simulink model "Tarea_1"  (R2013a)
settings: Solver=ode45  StartTime=0.0  StopTime=10  RelTol=1e-3
libraries: simulink x1
settings Model: Creator=Miguel  LastModifiedBy=Miguel

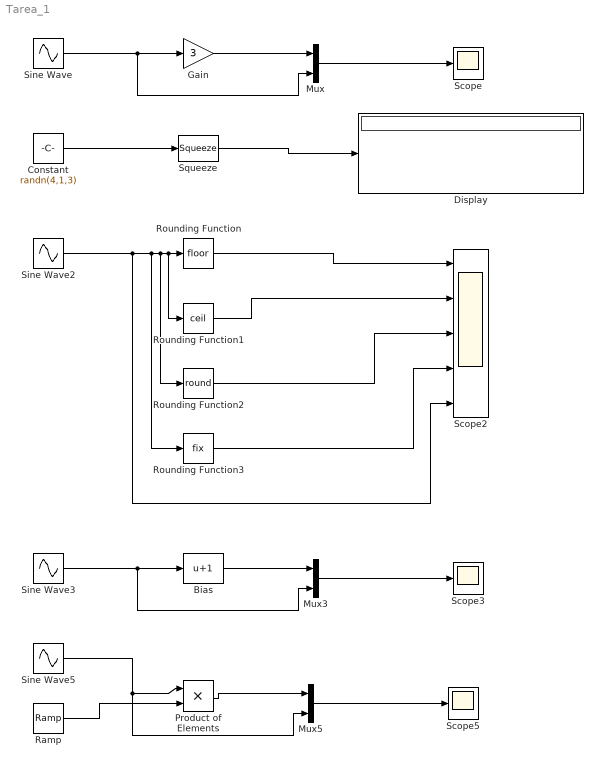
== system Tarea_1 ==
  Bias : Bias  Bias=1  SaturateOnIntegerOverflow=on
  Constant : Constant  Value=randn(4,1,3)  VectorParams1D=off
  Display : Display
  Gain : Gain  Gain=3
  Mux : Mux  Inputs=2
  Mux3 : Mux  Inputs=2
  Mux5 : Mux  Inputs=2
  Product of Elements : Product
  Ramp : simulink/Sources/Ramp  slope=1  start=0  X0=0
  Rounding Function : Rounding
  Rounding Function1 : Rounding  Operator=ceil
  Rounding Function2 : Rounding  Operator=round
  Rounding Function3 : Rounding  Operator=fix
  Scope : Scope
      settings: TickLabels=on
  Scope2 : Scope  NumInputPorts=5
      settings: TickLabels=on  YMin=-5~-5~-5~-5~-5  YMax=5~5~5~5~5  SaveName=ScopeData2
  Scope3 : Scope
      settings: TickLabels=on  SaveName=ScopeData3
  Scope5 : Scope
      settings: TickLabels=on  SaveName=ScopeData5
  Sine Wave : Sin  SampleTime=0
  Sine Wave2 : Sin  SampleTime=0
  Sine Wave3 : Sin  SampleTime=0
  Sine Wave5 : Sin  Frequency=10  SampleTime=0
  Squeeze : Squeeze
  wires:
  Gain/1 -> Mux/1
  Sine Wave/1 -> Mux/2, Gain/1
  Mux/1 -> Scope/1
  Rounding Function/1 -> Scope2/1
  Sine Wave2/1 -> Scope2/5, Rounding Function3/1, Rounding Function2/1, Rounding Function1/1, Rounding Function/1
  Sine Wave3/1 -> Bias/1, Mux3/2
  Mux3/1 -> Scope3/1
  Bias/1 -> Mux3/1
  Sine Wave5/1 -> Product of Elements/1, Mux5/2
  Mux5/1 -> Scope5/1
  Product of Elements/1 -> Mux5/1
  Squeeze/1 -> Display/1
  Constant/1 -> Squeeze/1
  Rounding Function1/1 -> Scope2/2
  Rounding Function2/1 -> Scope2/3
  Rounding Function3/1 -> Scope2/4
  Ramp/1 -> Product of Elements/2
